simulink model "FPGA_Comm_fpu_test"  (Simulink 7.6)
settings: Solver=ode4  StartTime=0.0  StopTime=inf  FixedStep=0.001  MaxStep=1e-1  RelTol=1e-3
settings Model: Creator=jordan  LastModifiedBy=jordan
settings GRTTargetCC: ExtMode=on

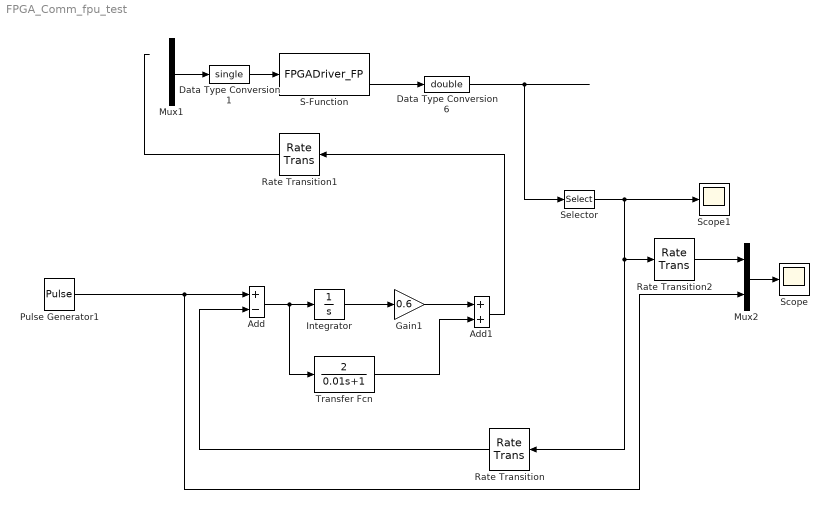
== system FPGA_Comm_fpu_test ==
  Add : Sum  Inputs=+-  SampleTime=0
  Add1 : Sum
  Data Type Conversion1 : DataTypeConversion  OutDataTypeStr=single
  Data Type Conversion6 : DataTypeConversion  OutDataTypeStr=double
  Gain1 : Gain  Gain=0.6
  Integrator : Integrator
  Mux1 : Mux  Inputs=2
  Mux2 : Mux  Inputs=2
  Pulse Generator1 : DiscretePulseGenerator  PulseType=Time based  Period=40  PulseWidth=50
  Rate Transition : RateTransition  Deterministic=off
  Rate Transition1 : RateTransition  Deterministic=off
  Rate Transition2 : RateTransition  Deterministic=off
  S-Function : S-Function  FunctionName=FPGADriver_FP  EnableBusSupport=off
  Scope : Scope
      settings: TimeRange=40  YMin=-0.2  YMax=1.1
  Scope1 : Scope
      settings: YMin=5.55112e-017  YMax=2
  Selector : Selector  InputPortWidth=2  IndexOptions=Index vector (dialog)  Indices=1  OutputSizes=1
  Transfer Fcn : TransferFcn  Numerator=[2]  Denominator=[0.01 1]
  wires:
  S-Function/2 -> Data Type Conversion6/1
  Data Type Conversion1/1 -> S-Function/1
  Mux1/1 -> Data Type Conversion1/1
  Data Type Conversion6/1 -> Selector/1
  Mux2/1 -> Scope/1
  Pulse Generator1/1 -> Mux2/2, Add/1
  Selector/1 -> Scope1/1, Rate Transition/1, Rate Transition2/1
  Add/1 -> Integrator/1, Transfer Fcn/1
  Integrator/1 -> Gain1/1
  Gain1/1 -> Add1/1
  Transfer Fcn/1 -> Add1/2
  Add1/1 -> Rate Transition1/1
  Rate Transition/1 -> Add/2
  Rate Transition1/1 -> ?
  Rate Transition2/1 -> Mux2/1
